simulink model "spacecraft_attitude_model"  (R2024b)
settings: Solver=ode4  StartTime=t0  StopTime=tf  FixedStep=0.1  RelTol=1e-3
values from neighbouring files (symbols this model uses):
  a = (((T/(2*pi))^2*mu_earth)^(1/3))    (= 7069867.85099)    [main_spacecraft_attitude_dynamics.m]
  A_body1 = surface(1)    [main_spacecraft_attitude_dynamics.m]
  A_body2 = surface(2)    [main_spacecraft_attitude_dynamics.m]
  A_body3 = surface(3)    [main_spacecraft_attitude_dynamics.m]
  A_body4 = surface(4)    [main_spacecraft_attitude_dynamics.m]
  A_body5 = surface(5)    [main_spacecraft_attitude_dynamics.m]
  A_body6 = surface(6)    [main_spacecraft_attitude_dynamics.m]
  A_panel1 = surface(7)    [main_spacecraft_attitude_dynamics.m]
  A_panel2 = surface(8)    [main_spacecraft_attitude_dynamics.m]
  A_panel3 = surface(9)    [main_spacecraft_attitude_dynamics.m]
  A_panel4 = surface(10)    [main_spacecraft_attitude_dynamics.m]
  alpha = [alpha1,alpha2,alpha3]    [main_spacecraft_attitude_dynamics.m]
  Ap = pinv(Ar)    [main_spacecraft_attitude_dynamics.m]
  Ar = Ar./norm(Ar)    [main_spacecraft_attitude_dynamics.m]
  AtmosphereModel = struct()    [AtmosphereData.m]    (also in main_spacecraft_attitude_dynamics.m)
  CD = 2.6    [main_spacecraft_attitude_dynamics.m]
  D_max = 50    [main_spacecraft_attitude_dynamics.m]
  Detumbling_time = 5000    [main_spacecraft_attitude_dynamics.m]
  e = 0.001    [main_spacecraft_attitude_dynamics.m]
  FOV = 128 * pi/180    (= 2.23402144255)    [main_spacecraft_attitude_dynamics.m]
  g1_0 = DGRF2020(1).g_nm    [main_spacecraft_attitude_dynamics.m]
  g1_1 = DGRF2020(2).g_nm    [main_spacecraft_attitude_dynamics.m]
  H = 700    [main_spacecraft_attitude_dynamics.m]
  h0 = 0    [main_spacecraft_attitude_dynamics.m]
  h1_1 = DGRF2020(2).h_nm    [main_spacecraft_attitude_dynamics.m]
  i = deg2rad(98.18)    [main_spacecraft_attitude_dynamics.m]
  Ir = 0.1    [main_spacecraft_attitude_dynamics.m]
  J = EXTRACTED_DATA.I_total    [main_spacecraft_attitude_dynamics.m]
  j_B = [0.01, 0.05, 0.01]'    [main_spacecraft_attitude_dynamics.m]
  k1 = max(max(kd_slew))    [main_spacecraft_attitude_dynamics.m]
  k2 = max(max(kp_slew))    [main_spacecraft_attitude_dynamics.m]
  Kw = max(max(kp_detumbling))    [main_spacecraft_attitude_dynamics.m]
  n = sqrt((G*M_E)/(r_earth^3))    [main_spacecraft_attitude_dynamics.m]
  N_B1 = N_B(1, :)'    [main_spacecraft_attitude_dynamics.m]
  N_B2 = N_B(2, :)'    [main_spacecraft_attitude_dynamics.m]
  N_B3 = N_B(3, :)'    [main_spacecraft_attitude_dynamics.m]
  N_B4 = N_B(4, :)'    [main_spacecraft_attitude_dynamics.m]
  N_B5 = N_B(5, :)'    [main_spacecraft_attitude_dynamics.m]
  N_B6 = N_B(6, :)'    [main_spacecraft_attitude_dynamics.m]
  N_P1 = N_B(7, :)'    [main_spacecraft_attitude_dynamics.m]
  N_P2 = N_B(8, :)'    [main_spacecraft_attitude_dynamics.m]
  N_P3 = N_B(9, :)'    [main_spacecraft_attitude_dynamics.m]
  N_P4 = N_B(10, :)'    [main_spacecraft_attitude_dynamics.m]
  n_S = (2*pi)/T_S    (= 1.99238499086e-07)    [main_spacecraft_attitude_dynamics.m]
  om = deg2rad(0)    [main_spacecraft_attitude_dynamics.m]
  P = Fe/c    (= 4.52980041279e-06)    [main_spacecraft_attitude_dynamics.m]
  pd_body1 = rho_D(1)    [main_spacecraft_attitude_dynamics.m]
  pd_body2 = rho_D(2)    [main_spacecraft_attitude_dynamics.m]
  pd_body3 = rho_D(3)    [main_spacecraft_attitude_dynamics.m]
  pd_body4 = rho_D(4)    [main_spacecraft_attitude_dynamics.m]
  pd_body5 = rho_D(5)    [main_spacecraft_attitude_dynamics.m]
  pd_body6 = rho_D(6)    [main_spacecraft_attitude_dynamics.m]
  pd_panel1 = rho_D(7)    [main_spacecraft_attitude_dynamics.m]
  pd_panel2 = rho_D(8)    [main_spacecraft_attitude_dynamics.m]
  pd_panel3 = rho_D(9)    [main_spacecraft_attitude_dynamics.m]
  pd_panel4 = rho_D(10)    [main_spacecraft_attitude_dynamics.m]
  ps_body1 = rho_S(1)    [main_spacecraft_attitude_dynamics.m]
  ps_body2 = rho_S(2)    [main_spacecraft_attitude_dynamics.m]
  ps_body3 = rho_S(3)    [main_spacecraft_attitude_dynamics.m]
  ps_body4 = rho_S(4)    [main_spacecraft_attitude_dynamics.m]
  ps_body5 = rho_S(5)    [main_spacecraft_attitude_dynamics.m]
  ps_body6 = rho_S(6)    [main_spacecraft_attitude_dynamics.m]
  ps_panel1 = rho_S(7)    [main_spacecraft_attitude_dynamics.m]
  ps_panel2 = rho_S(8)    [main_spacecraft_attitude_dynamics.m]
  ps_panel3 = rho_S(9)    [main_spacecraft_attitude_dynamics.m]
  ps_panel4 = rho_S(10)    [main_spacecraft_attitude_dynamics.m]
  q0 = [q1_0 q2_0 q3_0 q4_0]    [main_spacecraft_attitude_dynamics.m]
  r_earth = (R_earth + H)*10^3    (= 7078136.3)    [main_spacecraft_attitude_dynamics.m]
  R_earth = 6378.1363    [main_spacecraft_attitude_dynamics.m]
  r_f1 = r_F(1, :)'    [main_spacecraft_attitude_dynamics.m]
  r_f10 = r_F(10, :)'    [main_spacecraft_attitude_dynamics.m]
  r_f2 = r_F(2, :)'    [main_spacecraft_attitude_dynamics.m]
  r_f3 = r_F(3, :)'    [main_spacecraft_attitude_dynamics.m]
  r_f4 = r_F(4, :)'    [main_spacecraft_attitude_dynamics.m]
  r_f5 = r_F(5, :)'    [main_spacecraft_attitude_dynamics.m]
  r_f6 = r_F(6, :)'    [main_spacecraft_attitude_dynamics.m]
  r_f7 = r_F(7, :)'    [main_spacecraft_attitude_dynamics.m]
  r_f8 = r_F(8, :)'    [main_spacecraft_attitude_dynamics.m]
  r_f9 = r_F(9, :)'    [main_spacecraft_attitude_dynamics.m]
  r_Sun = 149597870    [main_spacecraft_attitude_dynamics.m]
  RAAN = deg2rad(RAAN)    [main_spacecraft_attitude_dynamics.m]
  sigma_b = RRW*(pi/180)*(1/3600)*(1/sqrt(Ts))    [main_spacecraft_attitude_dynamics.m]
  sigma_mag = 10^-6    (= 1e-06)    [main_spacecraft_attitude_dynamics.m]
  sigma_n = ARW*(pi/180)*(1/60)*(1/sqrt(Ts))    [main_spacecraft_attitude_dynamics.m]
  T_coil_max = 50 * 45*10^-6    (= 0.00225)    [main_spacecraft_attitude_dynamics.m]
  th0 = 0    [main_spacecraft_attitude_dynamics.m]
  v0 = [0 0 0]    [main_spacecraft_attitude_dynamics.m]
  variance_Ss = (a_sun)^2    (= 3.24)    [main_spacecraft_attitude_dynamics.m]
  w_0 = [-3, 3, 3]'    [main_spacecraft_attitude_dynamics.m]
  w_E = (2*pi)/(24*60*60)    (= 7.27220521664e-05)    [main_spacecraft_attitude_dynamics.m]
  w_LN = [0 0 0]'    [main_spacecraft_attitude_dynamics.m]
undefined symbols (not defined in the file or in its folder): A_Ss_orienation
libraries: matrix_library x38, slpidlib x2, aerolibutil x1, vrlib x1
(part 2 of 4)

== system spacecraft_attitude_model/Kinematics/quaternions to DCM ==
  note: Also here it should be A_NB 'cause we are going from
      | the inertial frame reference to the body one
  note: In reality it should be called A_BN but in the lab slides they call it in this way
  q : Inport
  To Workspace : ToWorkspace  VariableName=A_NB  SampleTime=-1
  q2A_DCM : Subsystem
  A_BN : Outport
  wires:
  q2A_DCM/1(A_NB) -> A_BN/1, To Workspace/1
  q/1 -> q2A_DCM/1(q)

== system spacecraft_attitude_model/Pointing error/DCM err (1) ==
  note: To wrap the acos
  A_ref : Inport
  Acos : Trigonometry  Operator=acos
  Constant : Constant
  Gain : Gain  Gain=180/pi
  Gain1 : Gain  Gain=0.5
  MATLAB Function : MATLAB Function  TreatAsAtomicUnit=on
  Saturation4 : Saturate  UpperLimit=1  LowerLimit=-1
  Sum : Sum  Inputs=-+|
  err : Outport
  wires:
  A_ref/1 -> MATLAB Function/1(A)
  Sum/1 -> Gain1/1
  Acos/1 -> Gain/1
  Constant/1 -> Sum/1
  Gain/1 -> err/1
  Gain1/1 -> Saturation4/1
  MATLAB Function/1(tr) -> Sum/2
  Saturation4/1 -> Acos/1

== system spacecraft_attitude_model/Pointing error/Subsystem1 ==
  note: q_BL = q_LN^-1 q_BN
  note: q_bn-1 q_LN v q_LN-1 q_BN
  q_BN_sensed : Inport
  q_LN : Inport  Port=2
  Gain1 : Gain  Gain=[-1; -1; -1; 1]
  Scope : Scope
  Scope1 : Scope
  Scope2 : Scope
  "q'' = q x q' " : Subsystem
  q_BL : Outport
  wires:
  "q'' = q x q' "/1(q'') -> q_BL/1  "q_BL"
  q_BN_sensed/1 -> Scope/1, "q'' = q x q' "/2(q')
  q_LN/1 -> Scope1/1, Gain1/1
  Gain1/1 -> Scope2/1, "q'' = q x q' "/1(q)  "q^-1"

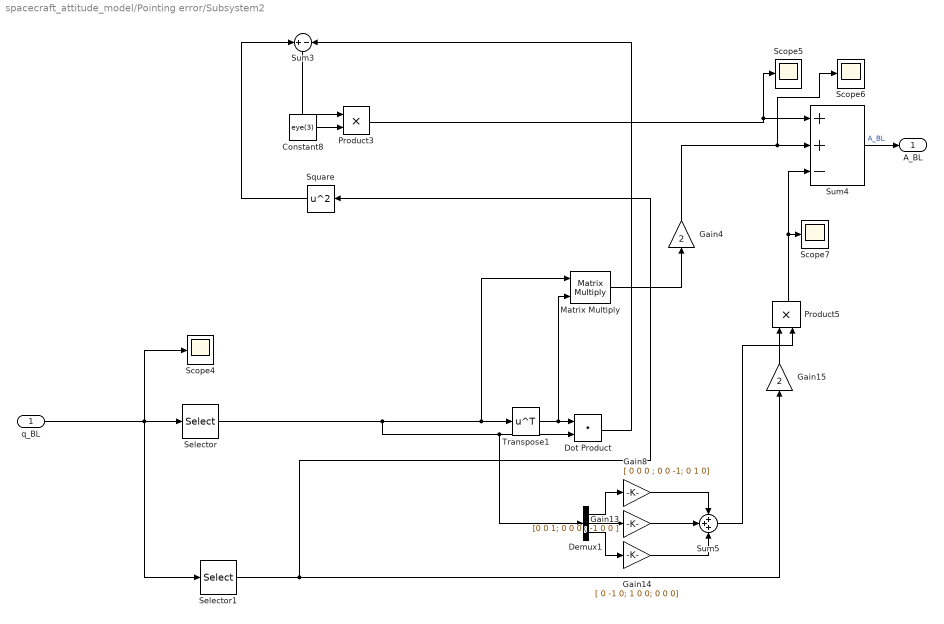
== system spacecraft_attitude_model/Pointing error/Subsystem2 ==
  q_BL : Inport
  Constant8 : Constant  Value=eye(3)
  Demux1 : Demux  Outputs=3
  Dot Product : DotProduct  OutDataTypeStr=Inherit: Inherit via internal rule
  Gain13 : Gain  Gain=[0 0 1; 0 0 0 ; -1 0 0 ]
  Gain14 : Gain  Gain=[ 0 -1 0; 1 0 0; 0 0 0]
  Gain15 : Gain  Gain=2
  Gain4 : Gain  Gain=2
  Gain8 : Gain  Gain=[ 0 0 0 ; 0 0 -1; 0 1 0]
  Matrix Multiply : Product  Multiplication=Matrix(*)
  Product3 : Product
  Product5 : Product
  Scope{4..7} (4 alike) : Scope
  Selector : Selector  NumberOfDimensions=2  InputPortWidth=3  IndexOptions=Index vector (dialog),Index vector (dialog)  Indices=[1 2 3],1  OutputSizes=1,1
  Selector1 : Selector  NumberOfDimensions=2  InputPortWidth=3  IndexOptions=Index vector (dialog),Index vector (dialog)  Indices=4,1  OutputSizes=1,1
  Square : Math  Operator=square
  Sum3 : Sum  Inputs=+-
  Sum4 : Sum  Inputs=++-
  Sum5 : Sum  Inputs=+++
  Transpose1 : Math  Operator=transpose
  A_BL : Outport
  wires:
  Constant8/1 -> Product3/2
  Matrix Multiply/1 -> Gain4/1
  Gain14/1 -> Sum5/3
  Product5/1 -> Scope7/1, Sum4/3
  Transpose1/1 -> Matrix Multiply/2, Dot Product/1
  Gain13/1 -> Sum5/2
  Sum5/1 -> Product5/2
  Gain8/1 -> Sum5/1
  Demux1/3 -> Gain14/1
  Sum4/1 -> A_BL/1  "A_BL"
  Product3/1 -> Scope5/1, Sum4/1
  Square/1 -> Sum3/1
  Selector/1 -> Matrix Multiply/1, Transpose1/1, Demux1/1, Dot Product/2
  Gain4/1 -> Scope6/1, Sum4/2
  Demux1/1 -> Gain8/1
  Gain15/1 -> Product5/1
  q_BL/1 -> Scope4/1, Selector/1, Selector1/1
  Sum3/1 -> Product3/1
  Dot Product/1 -> Sum3/2
  Selector1/1 -> Square/1, Gain15/1
  Demux1/2 -> Gain13/1

== system spacecraft_attitude_model/Pointing error/q_LN1 ==
  theta : Inport
  Constant : Constant  Value=[0; 0; 1]
  Constant1 : Constant  Value=[1; 0; 0]
  Constant2 : Constant  Value=i
  angle2quaternion : Subsystem
  angle2quaternion1 : Subsystem
  "q'' = q x q' " : Subsystem
  q_LN : Outport
  wires:
  theta/1 -> angle2quaternion/1(angle)
  Constant/1 -> angle2quaternion/2(e)
  Constant1/1 -> angle2quaternion1/2(e)
  Constant2/1 -> angle2quaternion1/1(angle)
  angle2quaternion1/1(q) -> "q'' = q x q' "/1(q)
  angle2quaternion/1(q) -> "q'' = q x q' "/2(q')
  "q'' = q x q' "/1(q'') -> q_LN/1

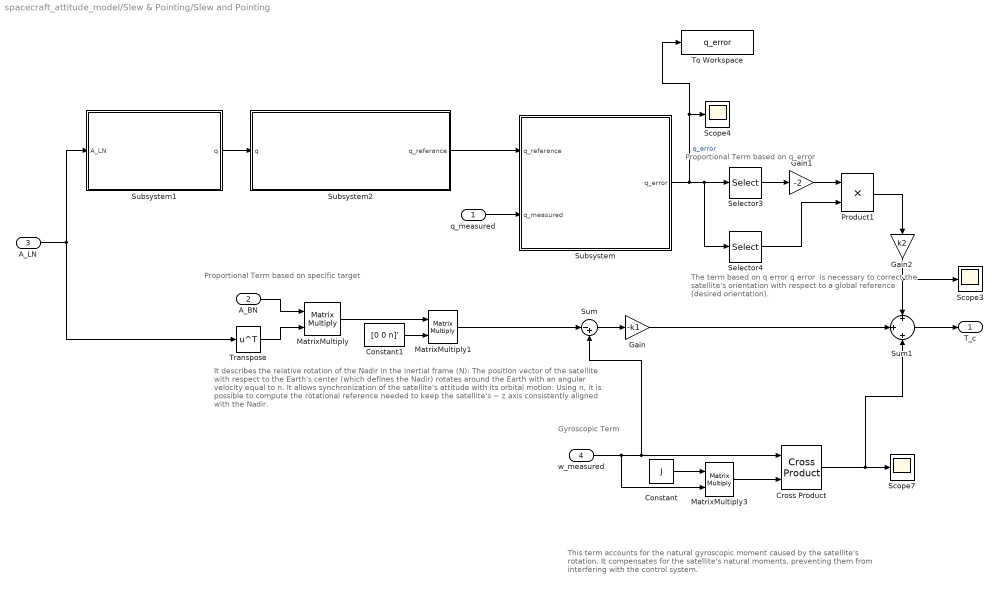
== system spacecraft_attitude_model/Slew & Pointing/Slew and Pointing ==
  note: The term based on q error q error ​ is necessary to correct the satellite's orientation with respect to a global reference (desired orientation).
  note: Proportional Term based on q_error
  note: This term accounts for the natural gyroscopic moment caused by the satellite's rotation. It compensates for the satellite's natural moments, preventing them from interfering with the control system.
  note: Proportional Term based on specific target
  note: It describes the relative rotation of the Nadir in the inertial frame (N): The position vector of the satellite with respect to the Earth's center (which defines the Nadir) rotates around the Earth with an angular velocity equal to n. It allows synchronization of the satellite's attitude with its orbital motion: Using n, it is possible to compute the rotational reference needed to keep the satellite's − z axis consistently aligned with the Nadir.
  note: Gyroscopic Term
  q_measured : Inport
  A_BN : Inport  Port=2
  A_LN : Inport  Port=3
  w_measured : Inport  Port=4
  Constant : Constant  Value=J
  Constant1 : Constant  Value=[0 0 n]'
  Cross Product : matrix_library/Cross Product
  Gain : Gain  Gain=-k1
  Gain1 : Gain  Gain=-2
  Gain2 : Gain  Gain=k2
  MatrixMultiply : Product  Multiplication=Matrix(*)
  MatrixMultiply1 : Product  Multiplication=Matrix(*)
  MatrixMultiply3 : Product  Multiplication=Matrix(*)
  Product1 : Product
  Scope3 : Scope
  Scope4 : Scope
  Scope7 : Scope
  Selector3 : Selector  InputPortWidth=4  IndexOptions=Index vector (dialog)  Indices=4  OutputSizes=1
  Selector4 : Selector  InputPortWidth=4  IndexOptions=Index vector (dialog)  Indices=[1:3]  OutputSizes=1
  Subsystem : Subsystem
  Subsystem1 : Subsystem
  Subsystem2 : Subsystem
  Sum : Sum  Inputs=|-+
  Sum1 : Sum  Inputs=+|+|+
  To Workspace : ToWorkspace  VariableName=q_error  SampleTime=-1
  Transpose : Math  Operator=transpose
  T_c : Outport
  wires:
  Transpose/1 -> MatrixMultiply/2
  MatrixMultiply/1 -> MatrixMultiply1/1
  w_measured/1 -> Sum/2, Cross Product/1, MatrixMultiply3/2
  Sum/1 -> Gain/1
  Gain/1 -> Sum1/2
  Constant/1 -> MatrixMultiply3/1
  MatrixMultiply3/1 -> Cross Product/2
  Cross Product/1 -> Scope7/1, Sum1/3
  Sum1/1 -> T_c/1
  q_measured/1 -> Subsystem/2(q_measured)
  Subsystem/1(q_error) -> Selector3/1, Selector4/1, To Workspace/1, Scope4/1  "q_error"
  Product1/1 -> Gain2/1
  Gain2/1 -> Sum1/1, Scope3/1
  Selector4/1 -> Product1/2
  Subsystem1/1(q) -> Subsystem2/1(q)
  A_BN/1 -> MatrixMultiply/1
  Subsystem2/1(q_referance) -> Subsystem/1(q_referance)
  Selector3/1 -> Gain1/1
  Gain1/1 -> Product1/1
  Constant1/1 -> MatrixMultiply1/2
  MatrixMultiply1/1 -> Sum/1
  A_LN/1 -> Subsystem1/1(A_LN), Transpose/1

== system spacecraft_attitude_model/Slew & Pointing/Subsystem ==
  b_measured : Inport
  T_control : Inport  Port=2
  w_measured : Inport  Port=3
  Constant : Constant  Value=Ar
  Inertia Wheel : Subsystem
  Magnetic coils : Subsystem
  Product : Product
  Scope : Scope  NumInputPorts=2
  Scope1 : Scope
  Subtract : Sum  Inputs=+-
  Sum : Sum  Inputs=|++
  To Workspace : ToWorkspace  VariableName=T_wheel_point1  SampleTime=-1
  T_act : Outport
  wires:
  Magnetic coils/1(T_coils) -> Sum/2
  Constant/1 -> Product/1
  Product/1 -> Subtract/2, Scope/1, Inertia Wheel/2(T_c_inertia)  "T_c_inertia"
  Inertia Wheel/1(T_wheel) -> To Workspace/1, Sum/1
  Sum/1 -> Scope1/1, T_act/1
  T_control/1 -> Product/2, Subtract/1
  Subtract/1 -> Magnetic coils/1(T_Control), Scope/2  "T_c_coils"
  b_measured/1 -> Magnetic coils/2(b_measured)
  w_measured/1 -> Inertia Wheel/1(w_measured)

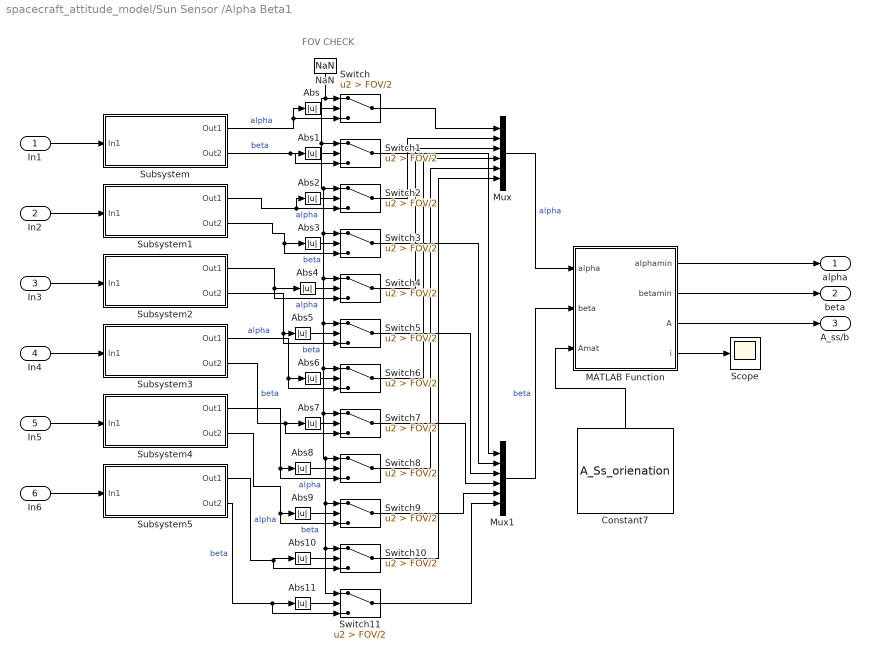
== system spacecraft_attitude_model/Sun Sensor /Alpha Beta1 ==
  note: FOV CHECK
  In1 : Inport
  In2 : Inport  Port=2
  In3 : Inport  Port=3
  In4 : Inport  Port=4
  In5 : Inport  Port=5
  In6 : Inport  Port=6
  Abs{,1..11} (12 alike) : Abs  SaturateOnIntegerOverflow=off
  Constant7 : Constant  Value=A_Ss_orienation
  MATLAB Function : MATLAB Function  TreatAsAtomicUnit=on
  Mux : Mux  Inputs=6
  Mux1 : Mux  Inputs=6
  NaN : Constant  Value=NaN  OutDataTypeStr=Inherit: Inherit via back propagation
  Scope : Scope
  Subsystem : Subsystem
  Subsystem1 : Subsystem
  Subsystem2 : Subsystem
  Subsystem3 : Subsystem
  Subsystem4 : Subsystem
  Subsystem5 : Subsystem
  Switch{,1..11} (12 alike) : Switch  Criteria=u2 > Threshold  Threshold=FOV/2  SaturateOnIntegerOverflow=off  InputSameDT=off
  alpha : Outport
  beta : Outport  Port=2
  A_ss/b : Outport  Port=3
  wires:
  Subsystem1/1(Out1) -> Abs2/1, Switch2/3  "alpha"
  Switch6/1 -> Mux/4
  Subsystem/2(Out2) -> Switch1/3, Abs1/1  "beta"
  In5/1 -> Subsystem4/1(In1)
  Abs10/1 -> Switch10/2
  Subsystem4/1(Out1) -> Switch8/3, Abs8/1  "alpha"
  Abs2/1 -> Switch2/2
  Subsystem2/1(Out1) -> Abs4/1, Switch4/3  "alpha"
  Subsystem3/1(Out1) -> Switch6/3, Abs6/1  "alpha"
  Switch1/1 -> Mux1/1
  Abs8/1 -> Switch8/2
  Switch5/1 -> Mux1/3
  Mux/1 -> MATLAB Function/1(alpha)  "alpha"
  Switch9/1 -> Mux1/5
  Subsystem2/2(Out2) -> Abs5/1, Switch5/3  "beta"
  Abs3/1 -> Switch3/2
  Subsystem1/2(Out2) -> Abs3/1, Switch3/3  "beta"
  Subsystem4/2(Out2) -> Switch9/3, Abs9/1  "beta"
  Switch11/1 -> Mux1/6
  Abs6/1 -> Switch6/2
  Switch3/1 -> Mux1/2
  Abs11/1 -> Switch11/2
  Abs1/1 -> Switch1/2
  In2/1 -> Subsystem1/1(In1)
  NaN/1 -> Switch11/1, Switch10/1, Switch9/1, Switch8/1, Switch7/1, Switch6/1, Switch5/1, Switch4/1, Switch3/1, Switch2/1, Switch1/1, Switch/1
  Subsystem/1(Out1) -> Abs/1, Switch/3  "alpha"
  Abs4/1 -> Switch4/2
  Subsystem3/2(Out2) -> Switch7/3, Abs7/1  "beta"
  Subsystem5/1(Out1) -> Switch10/3, Abs10/1  "alpha"
  Switch8/1 -> Mux/5
  Subsystem5/2(Out2) -> Abs11/1, Switch11/3  "beta"
  Switch7/1 -> Mux1/4
  In6/1 -> Subsystem5/1(In1)
  Abs9/1 -> Switch9/2
  Switch2/1 -> Mux/2
  Abs7/1 -> Switch7/2
  Abs5/1 -> Switch5/2
  Switch4/1 -> Mux/3
  Switch/1 -> Mux/1
  Abs/1 -> Switch/2
  Switch10/1 -> Mux/6
  In1/1 -> Subsystem/1(In1)
  Mux1/1 -> MATLAB Function/2(beta)  "beta"
  In4/1 -> Subsystem3/1(In1)
  In3/1 -> Subsystem2/1(In1)
  MATLAB Function/1(alphamin) -> alpha/1
  Constant7/1 -> MATLAB Function/3(Amat)
  MATLAB Function/4(i) -> Scope/1
  MATLAB Function/2(betamin) -> beta/1
  MATLAB Function/3(A) -> A_ss/b/1

== system spacecraft_attitude_model/Sun Sensor /Angle erros1 ==
  alpha_x : Inport
  alpha_y : Inport  Port=2
  alpha_z : Inport  Port=3
  Constant1 : Constant  Value=[1 0 0; 0 1 0; 0 0 1]
  Gain5 : Gain  Gain=[0 0 0; 0 0 1; 0 -1 0]
  Gain6 : Gain  Gain=[0 0 -1; 0 0 0; 1 0 0]
  Gain7 : Gain  Gain=[0 1 0; -1 0 0; 0 0 0]
  Sum : Sum  Inputs=|++++
  Out1 : Outport
  wires:
  Gain7/1 -> Sum/3
  alpha_y/1 -> Gain6/1
  Gain5/1 -> Sum/1
  alpha_x/1 -> Gain5/1
  Constant1/1 -> Sum/4
  Sum/1 -> Out1/1
  Gain6/1 -> Sum/2
  alpha_z/1 -> Gain7/1

== system spacecraft_attitude_model/Sun Sensor /Norm ==
  In1 : Inport
  Demux : Demux  Outputs=3
  Sqrt : Sqrt
  Square : Math  Operator=square
  Square1 : Math  Operator=square
  Square2 : Math  Operator=square
  Sum : Sum  Inputs=|+++
  Out1 : Outport
  wires:
  Demux/3 -> Square2/1
  In1/1 -> Demux/1
  Demux/1 -> Square/1
  Demux/2 -> Square1/1
  Square/1 -> Sum/1
  Square1/1 -> Sum/2
  Square2/1 -> Sum/3
  Sum/1 -> Sqrt/1
  Sqrt/1 -> Out1/1

== system spacecraft_attitude_model/Torque to w_dot_control/Torque to w_dot ==
  T_c : Inport
  Constant1 : Constant  Value=J
  Divide : Product  Inputs=*/  Multiplication=Matrix(*)
  "w_dot_control " : Outport
  wires:
  Divide/1 -> "w_dot_control "/1
  Constant1/1 -> Divide/2
  T_c/1 -> Divide/1

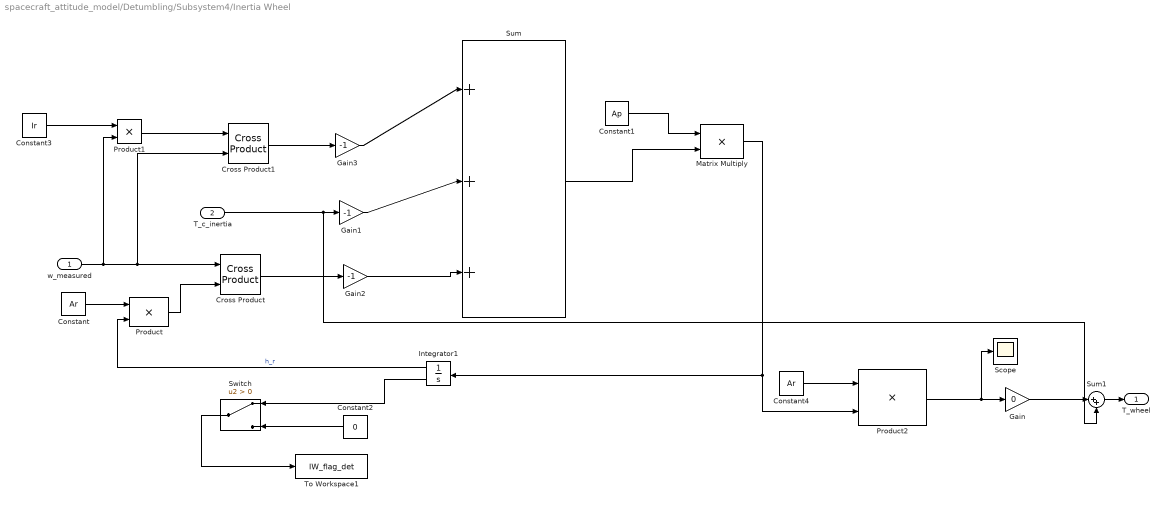
== system spacecraft_attitude_model/Detumbling/Subsystem4/Inertia Wheel ==
  w_measured : Inport
  T_c_inertia : Inport  Port=2
  Constant : Constant  Value=Ar
  Constant1 : Constant  Value=Ap
  Constant2 : Constant  Value=0
  Constant3 : Constant  Value=Ir
  Constant4 : Constant  Value=Ar
  Cross Product : matrix_library/Cross Product
  Cross Product1 : matrix_library/Cross Product
  Gain : Gain  Gain=0
  Gain1 : Gain  Gain=-1
  Gain2 : Gain  Gain=-1
  Gain3 : Gain  Gain=-1
  Integrator1 : Integrator  InitialCondition=h0  LimitOutput=on  UpperSaturationLimit=0.005  LowerSaturationLimit=-0.005  ShowSaturationPort=on
  Matrix Multiply : Product
  Product : Product
  Product1 : Product
  Product2 : Product
  Scope : Scope
  Sum : Sum  Inputs=|+++
  Sum1 : Sum  Inputs=|++
  Switch : Switch  Criteria=u2 > Threshold  SaturateOnIntegerOverflow=off  InputSameDT=off
  To Workspace1 : ToWorkspace  VariableName=IW_flag_det  SampleTime=-1
  T_wheel : Outport
  wires:
  Product/1 -> Cross Product/2
  Cross Product/1 -> Gain2/1
  w_measured/1 -> Product1/2, Cross Product1/2, Cross Product/1
  Gain2/1 -> Sum/3
  Constant1/1 -> Matrix Multiply/1
  Gain3/1 -> Sum/1
  Matrix Multiply/1 -> Product2/2, Integrator1/1
  Constant3/1 -> Product1/1
  Integrator1/1 -> Product/2  "h_r"
  Integrator1/2 -> Switch/1
  Constant2/1 -> Switch/3
  Constant/1 -> Product/1
  Product2/1 -> Scope/1, Gain/1
  Gain1/1 -> Sum/2
  Switch/1 -> To Workspace1/1
  Product1/1 -> Cross Product1/1
  Cross Product1/1 -> Gain3/1
  Constant4/1 -> Product2/1
  T_c_inertia/1 -> Sum1/2, Gain1/1
  Sum/1 -> Matrix Multiply/2
  Gain/1 -> Sum1/1
  Sum1/1 -> T_wheel/1

== system spacecraft_attitude_model/Detumbling/Subsystem4/Magnetic coils ==
  T_Control : Inport
  b_measured : Inport  Port=2
  Demux : Demux  Outputs=3
  Demux1 : Demux  Outputs=3
  Gain : Gain
  Gain1 : Gain
  Gain2 : Gain
  Norm1 : Subsystem
      settings: PortSchema="{\"entries\":[{\"content\":{\"sides\":[{\"content\":{},\"type\":\"ConnectorPlacement.EquallySpacedRectSide\",\"uuid\":\"c8e6b557-1f56-4290-9ece-bfc368650609\"},{\"content\":{\"connectorIds\":[\"Out1\"],\"side\":\"RIGHT\"},\"type\":\"ConnectorPlacement.EquallySpacedRectSide\",\"uuid\":\"77fa52b5-00ea-4466-8814-b89029d0f61f\"},{\"content\":{\"connectorIds\":[\"In1\"],\"side\":\"TOP\"},\"type\":\"ConnectorPlacement.EquallySpacedRectSide\",\"uuid\":\"5a1e965d-5eef-4834-963c-decfdd4da2be\"},{\"content\":{\"side\":\"BOTTOM\"},\"type\":\"ConnectorPlacement.EquallySpacedRectSide\",\"uuid\":\"d0b05173-3d81-4b7c-baba-8d47e4810e0f\"}]},\"type\":\"ConnectorPlacement.EquallySpacedConnector\",\"uuid\":\"bc13670f-664f-40fc-b4f3-9fab538d09d1\"}],\"packageUris\":[\"http://schema.mathworks.com/mf0/Connector/R2020b\"],\"version\":\"1.0\"}"
  Scope2 : Scope
  Square1 : Math  Operator=square
  Subsystem : Subsystem
  Subsystem1 : Subsystem
  Subsystem2 : Subsystem
  Vector Concatenate : Concatenate  NumInputs=3
  T_coils : Outport
  wires:
  Square1/1 -> Subsystem/3(b_norm^2), Subsystem1/3(b_norm^2), Subsystem2/3(b_norm^2)
  Demux1/2 -> Subsystem1/2(b_y)
  Demux/1 -> Gain/1
  Demux1/1 -> Subsystem/2(b_x)
  Gain1/1 -> Subsystem1/1(T_y)
  Gain/1 -> Subsystem/1(T_x)
  Gain2/1 -> Subsystem2/1(T_z)
  Demux1/3 -> Subsystem2/2(b_z)
  Demux/3 -> Gain2/1
  b_measured/1 -> Norm1/1(b), Demux1/1
  Norm1/1(b_norm) -> Square1/1  "b_norm"
  Demux/2 -> Gain1/1
  Vector Concatenate/1 -> T_coils/1, Scope2/1
  T_Control/1 -> Demux/1
  Subsystem2/1(T_coil_z) -> Vector Concatenate/3
  Subsystem1/1(T_coil_y) -> Vector Concatenate/2
  Subsystem/1(T_coil_x) -> Vector Concatenate/1

== system spacecraft_attitude_model/Disturbances Torque/Air Drag/A_Cross ==
  v_rB_versor : Inport
  A_CROSS1 : Subsystem
  A_CROSS10 : Subsystem
  A_CROSS2 : Subsystem
  A_CROSS3 : Subsystem
  A_CROSS4 : Subsystem
  A_CROSS5 : Subsystem
  A_CROSS6 : Subsystem
  A_CROSS7 : Subsystem
  A_CROSS8 : Subsystem
  A_CROSS9 : Subsystem
  A_cross1 : Outport
  A_cross2 : Outport  Port=2
  A_cross3 : Outport  Port=3
  A_cross4 : Outport  Port=4
  A_cross5 : Outport  Port=5
  A_cross6 : Outport  Port=6
  A_cross7 : Outport  Port=7
  A_cross8 : Outport  Port=8
  A_cross9 : Outport  Port=9
  A_cross10 : Outport  Port=10
  wires:
  A_CROSS5/1(A_cross2) -> A_cross5/1
  v_rB_versor/1 -> A_CROSS6/1(v_r_hat), A_CROSS7/1(v_r_hat), A_CROSS8/1(v_r_hat), A_CROSS9/1(v_r_hat), A_CROSS10/1(v_r_hat), A_CROSS5/1(v_r_hat), A_CROSS4/1(v_r_hat), A_CROSS3/1(v_r_hat), A_CROSS2/1(v_r_hat), A_CROSS1/1(v_r_hat)
  A_CROSS6/1(A_cross6) -> A_cross6/1
  A_CROSS4/1(A_cross4) -> A_cross4/1
  A_CROSS9/1(A_cross9) -> A_cross9/1
  A_CROSS2/1(A_cross2) -> A_cross2/1
  A_CROSS8/1(A_cross8) -> A_cross8/1
  A_CROSS3/1(A_cross3) -> A_cross3/1
  A_CROSS7/1(A_cross7) -> A_cross7/1
  A_CROSS10/1(A_cross10) -> A_cross10/1
  A_CROSS1/1(A_cross1) -> A_cross1/1

== system spacecraft_attitude_model/Disturbances Torque/Air Drag/Norm ==
  In1 : Inport
  Demux : Demux  Outputs=3
  Sqrt : Sqrt
  Square : Math  Operator=square
  Square1 : Math  Operator=square
  Square2 : Math  Operator=square
  Sum : Sum  Inputs=|+++
  v_rB_norm : Outport
  wires:
  Demux/3 -> Square2/1
  In1/1 -> Demux/1
  Demux/1 -> Square/1
  Demux/2 -> Square1/1
  Square/1 -> Sum/1
  Square1/1 -> Sum/2
  Square2/1 -> Sum/3
  Sum/1 -> Sqrt/1
  Sqrt/1 -> v_rB_norm/1

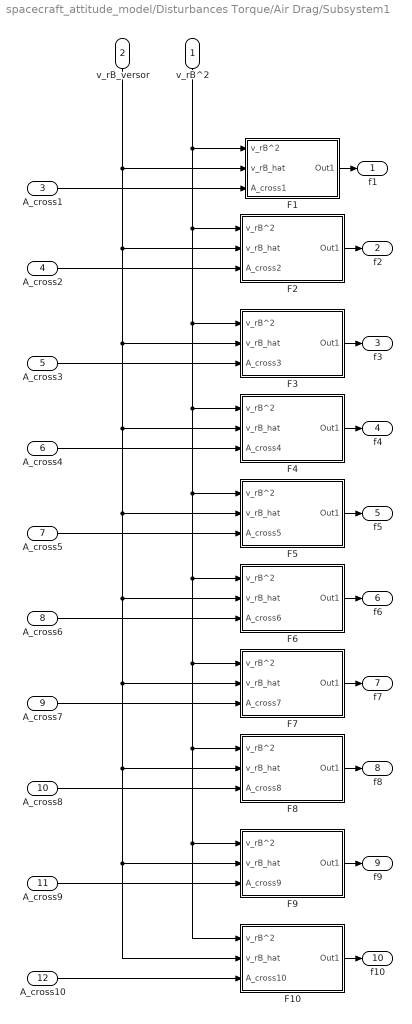
== system spacecraft_attitude_model/Disturbances Torque/Air Drag/Subsystem1 ==
  v_rB^2 : Inport
  v_rB_versor : Inport  Port=2
  A_cross1 : Inport  Port=3
  A_cross2 : Inport  Port=4
  A_cross3 : Inport  Port=5
  A_cross4 : Inport  Port=6
  A_cross5 : Inport  Port=7
  A_cross6 : Inport  Port=8
  A_cross7 : Inport  Port=9
  A_cross8 : Inport  Port=10
  A_cross9 : Inport  Port=11
  A_cross10 : Inport  Port=12
  F1 : Subsystem
  F10 : Subsystem
  F2 : Subsystem
  F3 : Subsystem
  F4 : Subsystem
  F5 : Subsystem
  F6 : Subsystem
  F7 : Subsystem
  F8 : Subsystem
  F9 : Subsystem
  f1 : Outport
  f2 : Outport  Port=2
  f3 : Outport  Port=3
  f4 : Outport  Port=4
  f5 : Outport  Port=5
  f6 : Outport  Port=6
  f7 : Outport  Port=7
  f8 : Outport  Port=8
  f9 : Outport  Port=9
  f10 : Outport  Port=10
  wires:
  v_rB^2/1 -> F1/1(v_rB^2), F2/1(v_rB^2), F3/1(v_rB^2), F4/1(v_rB^2), F5/1(v_rB^2), F6/1(v_rB^2), F7/1(v_rB^2), F8/1(v_rB^2), F9/1(v_rB^2), F10/1(v_rB^2)
  A_cross6/1 -> F6/3(A_cross6)
  v_rB_versor/1 -> F1/2(v_rB_hat), F2/2(v_rB_hat), F3/2(v_rB_hat), F4/2(v_rB_hat), F5/2(v_rB_hat), F6/2(v_rB_hat), F7/2(v_rB_hat), F8/2(v_rB_hat), F9/2(v_rB_hat), F10/2(v_rB_hat)
  A_cross5/1 -> F5/3(A_cross5)
  F5/1(Out1) -> f5/1
  A_cross4/1 -> F4/3(A_cross4)
  A_cross3/1 -> F3/3(A_cross3)
  A_cross9/1 -> F9/3(A_cross9)
  A_cross1/1 -> F1/3(A_cross1)
  F10/1(Out1) -> f10/1
  F7/1(Out1) -> f7/1
  A_cross8/1 -> F8/3(A_cross8)
  F6/1(Out1) -> f6/1
  F2/1(Out1) -> f2/1
  F3/1(Out1) -> f3/1
  F8/1(Out1) -> f8/1
  F1/1(Out1) -> f1/1
  A_cross10/1 -> F10/3(A_cross10)
  F4/1(Out1) -> f4/1
  F9/1(Out1) -> f9/1
  A_cross7/1 -> F7/3(A_cross7)
  A_cross2/1 -> F2/3(A_cross2)

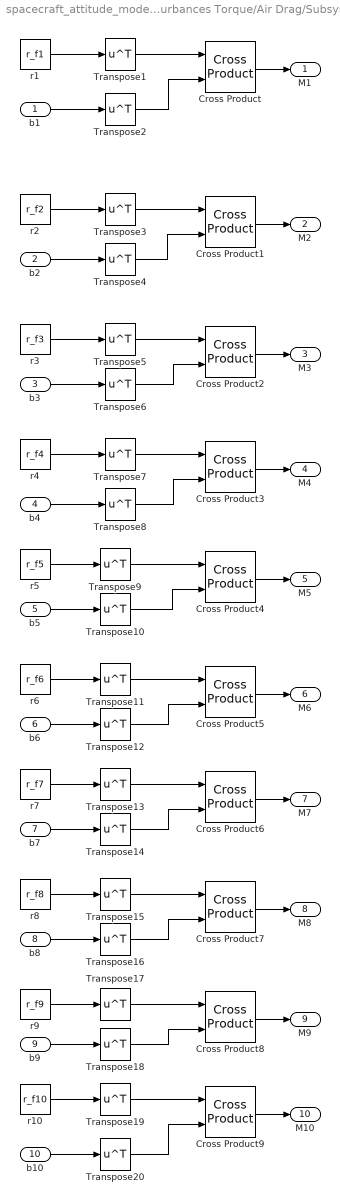
== system spacecraft_attitude_model/Disturbances Torque/Air Drag/Subsystem2 ==
  b1 : Inport
  b2 : Inport  Port=2
  b3 : Inport  Port=3
  b4 : Inport  Port=4
  b5 : Inport  Port=5
  b6 : Inport  Port=6
  b7 : Inport  Port=7
  b8 : Inport  Port=8
  b9 : Inport  Port=9
  b10 : Inport  Port=10
  Cross Product{,1..9} (10 alike) : matrix_library/Cross Product
  Transpose{1..20} (20 alike) : Math  Operator=transpose
  r1 : Constant  Value=r_f1
  r10 : Constant  Value=r_f10
  r2 : Constant  Value=r_f2
  r3 : Constant  Value=r_f3
  r4 : Constant  Value=r_f4
  r5 : Constant  Value=r_f5
  r6 : Constant  Value=r_f6
  r7 : Constant  Value=r_f7
  r8 : Constant  Value=r_f8
  r9 : Constant  Value=r_f9
  M1 : Outport
  M2 : Outport  Port=2
  M3 : Outport  Port=3
  M4 : Outport  Port=4
  M5 : Outport  Port=5
  M6 : Outport  Port=6
  M7 : Outport  Port=7
  M8 : Outport  Port=8
  M9 : Outport  Port=9
  M10 : Outport  Port=10
  wires:
  r1/1 -> Transpose1/1
  r10/1 -> Transpose19/1
  Cross Product8/1 -> M9/1
  r2/1 -> Transpose3/1
  Cross Product6/1 -> M7/1
  r6/1 -> Transpose11/1
  r5/1 -> Transpose9/1
  r9/1 -> Transpose17/1
  r7/1 -> Transpose13/1
  r4/1 -> Transpose7/1
  r8/1 -> Transpose15/1
  b6/1 -> Transpose12/1
  b2/1 -> Transpose4/1
  r3/1 -> Transpose5/1
  b1/1 -> Transpose2/1
  Cross Product3/1 -> M4/1
  b8/1 -> Transpose16/1
  Cross Product1/1 -> M2/1
  b5/1 -> Transpose10/1
  Cross Product7/1 -> M8/1
  b3/1 -> Transpose6/1
  Cross Product4/1 -> M5/1
  Cross Product2/1 -> M3/1
  Cross Product/1 -> M1/1
  Cross Product5/1 -> M6/1
  b10/1 -> Transpose20/1
  Cross Product9/1 -> M10/1
  b9/1 -> Transpose18/1
  b7/1 -> Transpose14/1
  b4/1 -> Transpose8/1
  Transpose1/1 -> Cross Product/1
  Transpose2/1 -> Cross Product/2
  Transpose3/1 -> Cross Product1/1
  Transpose4/1 -> Cross Product1/2
  Transpose5/1 -> Cross Product2/1
  Transpose6/1 -> Cross Product2/2
  Transpose7/1 -> Cross Product3/1
  Transpose8/1 -> Cross Product3/2
  Transpose9/1 -> Cross Product4/1
  Transpose10/1 -> Cross Product4/2
  Transpose11/1 -> Cross Product5/1
  Transpose12/1 -> Cross Product5/2
  Transpose13/1 -> Cross Product6/1
  Transpose14/1 -> Cross Product6/2
  Transpose15/1 -> Cross Product7/1
  Transpose16/1 -> Cross Product7/2
  Transpose17/1 -> Cross Product8/1
  Transpose18/1 -> Cross Product8/2
  Transpose19/1 -> Cross Product9/1
  Transpose20/1 -> Cross Product9/2

== system spacecraft_attitude_model/Disturbances Torque/Gravity Gradient/Gravity Gradient ==
  A_BL : Inport
  -3*n^2 : Gain  Gain=-3*(n^2)
  Constant4 : Constant  Value=J
  Constant5 : Constant  Value=inv(J)
  Cross Product2 : matrix_library/Cross Product
  Matrix Multiply : Product  Multiplication=Matrix(*)
  Matrix Multiply1 : Product  Multiplication=Matrix(*)
  c : Subsystem
  w_dot_GG : Outport
  wires:
  Constant5/1 -> Matrix Multiply1/1
  Cross Product2/1 -> Matrix Multiply1/2  "(Jc x c)"
  Matrix Multiply1/1 -> -3*n^2/1
  Matrix Multiply/1 -> Cross Product2/1
  Constant4/1 -> Matrix Multiply/1
  c/1(c) -> Cross Product2/2, Matrix Multiply/2
  A_BL/1 -> c/1(A_BL)
  -3*n^2/1 -> w_dot_GG/1

== system spacecraft_attitude_model/Disturbances Torque/Gravity Gradient/w_dot to torque ==
  w : Inport
  w_dot_GG : Inport  Port=2
  Constant : Constant  Value=J
  Cross Product : matrix_library/Cross Product
  Product : Product  Multiplication=Matrix(*)
  Transpose2 : Math  Operator=transpose
  Transpose3 : Math  Operator=transpose
  T_GG : Outport
  wires:
  Constant/1 -> Product/1
  w_dot_GG/1 -> Transpose2/1
  Product/1 -> Transpose3/1
  Cross Product/1 -> T_GG/1
  w/1 -> Product/2
  Transpose2/1 -> Cross Product/1
  Transpose3/1 -> Cross Product/2

== system spacecraft_attitude_model/Disturbances Torque/Solar_Radiation_Torque/Norm ==
  In1 : Inport
  Demux : Demux  Outputs=3
  Sqrt : Sqrt
  Square : Math  Operator=square
  Square1 : Math  Operator=square
  Square2 : Math  Operator=square
  Sum : Sum  Inputs=|+++
  Out1 : Outport
  wires:
  Demux/3 -> Square2/1
  In1/1 -> Demux/1
  Demux/1 -> Square/1
  Demux/2 -> Square1/1
  Square/1 -> Sum/1
  Square1/1 -> Sum/2
  Square2/1 -> Sum/3
  Sum/1 -> Sqrt/1
  Sqrt/1 -> Out1/1

== system spacecraft_attitude_model/Disturbances Torque/Solar_Radiation_Torque/SQR Force body 10 ==
  norm S_B : Inport
  -P*A : Gain  Gain=-P * A_panel4
  Constant : Constant  Value=N_P4
  Constant1 : Constant  Value=pd_panel4 * 2/3
  Constant2 : Constant  Value=0
  Constant3 : Constant  Value=r_f10
  Cross Product : matrix_library/Cross Product
  Dot Product : DotProduct  OutDataTypeStr=Inherit: Inherit via internal rule
  Gain1 : Gain  Gain=2*ps_panel4
  Gain2 : Gain  Gain=N_P4
  Gain3 : Gain  Gain=1-ps_panel4
  Product : Product
  Sum : Sum  Inputs=|++
  Sum1 : Sum  Inputs=|++
  Switch : Switch  Criteria=u2 > Threshold  SaturateOnIntegerOverflow=off  InputSameDT=off
  To Workspace : ToWorkspace  VariableName=T10  SampleTime=-1
  T10 : Outport
  wires:
  Gain2/1 -> Sum1/1
  Dot Product/1 -> Switch/2, Gain1/1, -P*A/1
  Switch/1 -> To Workspace/1, T10/1
  Product/1 -> Cross Product/2
  -P*A/1 -> Product/1
  Constant3/1 -> Cross Product/1
  Constant2/1 -> Switch/3
  Constant/1 -> Dot Product/2
  Sum/1 -> Gain2/1
  Gain3/1 -> Sum1/2
  Cross Product/1 -> Switch/1
  norm S_B/1 -> Gain3/1, Dot Product/1
  Sum1/1 -> Product/2
  Gain1/1 -> Sum/1
  Constant1/1 -> Sum/2

== system spacecraft_attitude_model/Disturbances Torque/Solar_Radiation_Torque/SQR Force body 6 ==
  norm S_B : Inport
  -P*A : Gain  Gain=-P * A_body6
  Constant : Constant  Value=N_B6
  Constant1 : Constant  Value=pd_body6 * 2/3
  Constant2 : Constant  Value=0
  Constant3 : Constant  Value=r_f6
  Cross Product : matrix_library/Cross Product
  Dot Product : DotProduct  OutDataTypeStr=Inherit: Inherit via internal rule
  Gain1 : Gain  Gain=2*ps_body6
  Gain2 : Gain  Gain=N_B6
  Gain3 : Gain  Gain=1-ps_body6
  Product : Product
  Sum : Sum  Inputs=|++
  Sum1 : Sum  Inputs=|++
  Switch : Switch  Criteria=u2 > Threshold  SaturateOnIntegerOverflow=off  InputSameDT=off
  To Workspace : ToWorkspace  VariableName=T6  SampleTime=-1
  T6 : Outport
  wires:
  Gain1/1 -> Sum/1
  Switch/1 -> To Workspace/1, T6/1
  -P*A/1 -> Product/1
  Constant1/1 -> Sum/2
  Constant/1 -> Dot Product/2
  Constant2/1 -> Switch/3
  norm S_B/1 -> Gain3/1, Dot Product/1
  Sum1/1 -> Product/2
  Cross Product/1 -> Switch/1
  Gain3/1 -> Sum1/2
  Sum/1 -> Gain2/1
  Dot Product/1 -> Switch/2, Gain1/1, -P*A/1
  Gain2/1 -> Sum1/1
  Product/1 -> Cross Product/2
  Constant3/1 -> Cross Product/1

== system spacecraft_attitude_model/Disturbances Torque/Solar_Radiation_Torque/SQR Force body 7 ==
  norm S_B : Inport
  -P*A : Gain  Gain=-P * A_panel1
  Constant : Constant  Value=N_P1
  Constant1 : Constant  Value=pd_panel1 * 2/3
  Constant2 : Constant  Value=0
  Constant3 : Constant  Value=r_f7
  Cross Product : matrix_library/Cross Product
  Dot Product : DotProduct  OutDataTypeStr=Inherit: Inherit via internal rule
  Gain1 : Gain  Gain=2*ps_panel1
  Gain2 : Gain  Gain=N_P1
  Gain3 : Gain  Gain=1-ps_panel1
  Product : Product
  Scope : Scope
  Sum : Sum  Inputs=|++
  Sum1 : Sum  Inputs=|++
  Switch : Switch  Criteria=u2 > Threshold  SaturateOnIntegerOverflow=off  InputSameDT=off
  To Workspace : ToWorkspace  VariableName=T7  SampleTime=-1
  T7 : Outport
  wires:
  Gain1/1 -> Sum/1
  Switch/1 -> To Workspace/1, Scope/1, T7/1
  -P*A/1 -> Product/1
  Constant1/1 -> Sum/2
  Constant/1 -> Dot Product/2
  Constant2/1 -> Switch/3
  norm S_B/1 -> Gain3/1, Dot Product/1
  Sum1/1 -> Product/2
  Cross Product/1 -> Switch/1
  Gain3/1 -> Sum1/2
  Sum/1 -> Gain2/1
  Dot Product/1 -> Switch/2, Gain1/1, -P*A/1
  Gain2/1 -> Sum1/1
  Product/1 -> Cross Product/2
  Constant3/1 -> Cross Product/1

== system spacecraft_attitude_model/Disturbances Torque/Solar_Radiation_Torque/SQR Force body 8 ==
  norm S_B : Inport
  -P*A : Gain  Gain=-P * A_panel2
  Constant : Constant  Value=N_P2
  Constant1 : Constant  Value=pd_panel2 * 2/3
  Constant2 : Constant  Value=0
  Constant3 : Constant  Value=r_f8
  Cross Product : matrix_library/Cross Product
  Dot Product : DotProduct  OutDataTypeStr=Inherit: Inherit via internal rule
  Gain1 : Gain  Gain=2*ps_panel2
  Gain2 : Gain  Gain=N_P2
  Gain3 : Gain  Gain=1-ps_panel2
  Product : Product
  Scope : Scope
  Sum : Sum  Inputs=|++
  Sum1 : Sum  Inputs=|++
  Switch : Switch  Criteria=u2 > Threshold  SaturateOnIntegerOverflow=off  InputSameDT=off
  To Workspace : ToWorkspace  VariableName=T8  SampleTime=-1
  T8 : Outport
  wires:
  Gain2/1 -> Sum1/1
  Dot Product/1 -> Switch/2, Gain1/1, -P*A/1
  Switch/1 -> To Workspace/1, Scope/1, T8/1
  Product/1 -> Cross Product/2
  -P*A/1 -> Product/1
  Constant3/1 -> Cross Product/1
  Constant2/1 -> Switch/3
  Constant/1 -> Dot Product/2
  Sum/1 -> Gain2/1
  Gain3/1 -> Sum1/2
  Cross Product/1 -> Switch/1
  norm S_B/1 -> Gain3/1, Dot Product/1
  Sum1/1 -> Product/2
  Gain1/1 -> Sum/1
  Constant1/1 -> Sum/2

== system spacecraft_attitude_model/Disturbances Torque/Solar_Radiation_Torque/SQR Force body 9 ==
  norm S_B : Inport
  -P*A : Gain  Gain=-P * A_panel3
  Constant : Constant  Value=N_P3
  Constant1 : Constant  Value=pd_panel3 * 2/3
  Constant2 : Constant  Value=0
  Constant3 : Constant  Value=r_f9
  Cross Product : matrix_library/Cross Product
  Dot Product : DotProduct  OutDataTypeStr=Inherit: Inherit via internal rule
  Gain1 : Gain  Gain=2*ps_panel3
  Gain2 : Gain  Gain=N_P3
  Gain3 : Gain  Gain=1-ps_panel3
  Product : Product
  Scope : Scope
  Sum : Sum  Inputs=|++
  Sum1 : Sum  Inputs=|++
  Switch : Switch  Criteria=u2 > Threshold  SaturateOnIntegerOverflow=off  InputSameDT=off
  To Workspace : ToWorkspace  VariableName=T9  SampleTime=-1
  T9 : Outport
  wires:
  Gain2/1 -> Sum1/1
  Dot Product/1 -> Switch/2, Gain1/1, -P*A/1
  Switch/1 -> To Workspace/1, Scope/1, T9/1
  Product/1 -> Cross Product/2
  -P*A/1 -> Product/1
  Constant3/1 -> Cross Product/1
  Constant2/1 -> Switch/3
  Constant/1 -> Dot Product/2
  Sum/1 -> Gain2/1
  Gain3/1 -> Sum1/2
  Cross Product/1 -> Switch/1
  norm S_B/1 -> Gain3/1, Dot Product/1
  Sum1/1 -> Product/2
  Gain1/1 -> Sum/1
  Constant1/1 -> Sum/2

== system spacecraft_attitude_model/Disturbances Torque/Solar_Radiation_Torque/SQR Torque body 4 ==
  norm S_B : Inport
  -P*A : Gain  Gain=-P*A_body4
  Constant : Constant  Value=N_B4
  Constant1 : Constant  Value=pd_body4 * 2/3
  Constant2 : Constant  Value=0
  Constant3 : Constant  Value=r_f4
  Cross Product : matrix_library/Cross Product
  Dot Product : DotProduct  OutDataTypeStr=Inherit: Inherit via internal rule
  Gain1 : Gain  Gain=2*ps_body4
  Gain2 : Gain  Gain=N_B4
  Gain3 : Gain  Gain=1-ps_body4
  Product : Product
  Sum : Sum  Inputs=|++
  Sum1 : Sum  Inputs=|++
  Switch : Switch  Criteria=u2 > Threshold  SaturateOnIntegerOverflow=off  InputSameDT=off
  To Workspace : ToWorkspace  VariableName=T4  SampleTime=-1
  T4 : Outport
  wires:
  Product/1 -> Cross Product/2
  Sum/1 -> Gain2/1
  norm S_B/1 -> Gain3/1, Dot Product/1
  Constant3/1 -> Cross Product/1
  Gain2/1 -> Sum1/1
  Gain1/1 -> Sum/1
  Constant1/1 -> Sum/2
  Sum1/1 -> Product/2
  Switch/1 -> To Workspace/1, T4/1
  Gain3/1 -> Sum1/2
  Constant2/1 -> Switch/3
  Cross Product/1 -> Switch/1
  -P*A/1 -> Product/1
  Dot Product/1 -> Switch/2, Gain1/1, -P*A/1
  Constant/1 -> Dot Product/2

== system spacecraft_attitude_model/Disturbances Torque/Solar_Radiation_Torque/SQR Torque body 5 ==
  norm S_B : Inport
  -P*A : Gain  Gain=-P * A_body5
  Constant : Constant  Value=N_B5
  Constant1 : Constant  Value=pd_body5 * 2/3
  Constant2 : Constant  Value=0
  Constant3 : Constant  Value=r_f5
  Cross Product : matrix_library/Cross Product
  Dot Product : DotProduct  OutDataTypeStr=Inherit: Inherit via internal rule
  Gain1 : Gain  Gain=2*ps_body5
  Gain2 : Gain  Gain=N_B5
  Gain3 : Gain  Gain=1-ps_body5
  Product : Product
  Sum : Sum  Inputs=|++
  Sum1 : Sum  Inputs=|++
  Switch : Switch  Criteria=u2 > Threshold  SaturateOnIntegerOverflow=off  InputSameDT=off
  To Workspace : ToWorkspace  VariableName=T5  SampleTime=-1
  T5 : Outport
  wires:
  Product/1 -> Cross Product/2
  Sum/1 -> Gain2/1
  norm S_B/1 -> Gain3/1, Dot Product/1
  Constant3/1 -> Cross Product/1
  Gain2/1 -> Sum1/1
  Gain1/1 -> Sum/1
  Constant1/1 -> Sum/2
  Sum1/1 -> Product/2
  Switch/1 -> To Workspace/1, T5/1
  Gain3/1 -> Sum1/2
  Constant2/1 -> Switch/3
  Cross Product/1 -> Switch/1
  -P*A/1 -> Product/1
  Dot Product/1 -> Switch/2, Gain1/1, -P*A/1
  Constant/1 -> Dot Product/2

== system spacecraft_attitude_model/Disturbances Torque/Solar_Radiation_Torque/SQR torque body 1 ==
  note: Switch: If the body is not illuminated
      | T = 0, in fact <0
  norm S_B : Inport
  -P*A : Gain  Gain=-P*A_body1
  Constant : Constant  Value=N_B1
  Constant1 : Constant  Value=pd_body1 * 2/3
  Constant2 : Constant  Value=0
  Constant3 : Constant  Value=r_f1
  Cross Product : matrix_library/Cross Product
  Dot Product : DotProduct  OutDataTypeStr=Inherit: Inherit via internal rule
  Gain1 : Gain  Gain=2*ps_body1
  Gain2 : Gain  Gain=N_B1
  Gain3 : Gain  Gain=1-ps_body1
  Product : Product
  Scope : Scope
  Sum : Sum  Inputs=|++
  Sum1 : Sum  Inputs=|++
  Switch : Switch  Criteria=u2 > Threshold  SaturateOnIntegerOverflow=off  InputSameDT=off
  To Workspace : ToWorkspace  VariableName=T1  SampleTime=-1
  T1 : Outport
  wires:
  norm S_B/1 -> Gain3/1, Dot Product/1
  Constant/1 -> Dot Product/2
  Dot Product/1 -> Switch/2, Gain1/1, -P*A/1
  Gain1/1 -> Sum/1
  Constant1/1 -> Sum/2
  Sum/1 -> Gain2/1
  Gain2/1 -> Sum1/1
  Gain3/1 -> Sum1/2
  -P*A/1 -> Product/1
  Sum1/1 -> Product/2
  Switch/1 -> To Workspace/1, Scope/1, T1/1
  Constant2/1 -> Switch/3
  Product/1 -> Cross Product/2
  Cross Product/1 -> Switch/1
  Constant3/1 -> Cross Product/1

== system spacecraft_attitude_model/Disturbances Torque/Solar_Radiation_Torque/SQR torque body 3 ==
  norm S_B : Inport
  -P*A : Gain  Gain=-P*A_body3
  Constant : Constant  Value=N_B3
  Constant1 : Constant  Value=pd_body3 * 2/3
  Constant2 : Constant  Value=0
  Constant3 : Constant  Value=r_f3
  Cross Product : matrix_library/Cross Product
  Dot Product : DotProduct  OutDataTypeStr=Inherit: Inherit via internal rule
  Gain1 : Gain  Gain=2*ps_body3
  Gain2 : Gain  Gain=N_B3
  Gain3 : Gain  Gain=1-ps_body3
  Product : Product
  Sum : Sum  Inputs=|++
  Sum1 : Sum  Inputs=|++
  Switch : Switch  Criteria=u2 > Threshold  SaturateOnIntegerOverflow=off  InputSameDT=off
  To Workspace : ToWorkspace  VariableName=T3  SampleTime=-1
  T3 : Outport
  wires:
  Product/1 -> Cross Product/2
  Sum/1 -> Gain2/1
  norm S_B/1 -> Gain3/1, Dot Product/1
  Constant3/1 -> Cross Product/1
  Gain2/1 -> Sum1/1
  Gain1/1 -> Sum/1
  Constant1/1 -> Sum/2
  Sum1/1 -> Product/2
  Switch/1 -> To Workspace/1, T3/1
  Gain3/1 -> Sum1/2
  Constant2/1 -> Switch/3
  Cross Product/1 -> Switch/1
  -P*A/1 -> Product/1
  Dot Product/1 -> Switch/2, Gain1/1, -P*A/1
  Constant/1 -> Dot Product/2

== system spacecraft_attitude_model/Disturbances Torque/Solar_Radiation_Torque/SQR torquw body 2 ==
  norm S_B : Inport
  -P*A : Gain  Gain=-P*A_body2
  Constant : Constant  Value=N_B2
  Constant1 : Constant  Value=pd_body2 * 2/3
  Constant2 : Constant  Value=0
  Constant3 : Constant  Value=r_f2
  Cross Product : matrix_library/Cross Product
  Dot Product : DotProduct  OutDataTypeStr=Inherit: Inherit via internal rule
  Gain1 : Gain  Gain=2*ps_body2
  Gain2 : Gain  Gain=N_B2
  Gain3 : Gain  Gain=1-ps_body2
  Product : Product
  Sum : Sum  Inputs=|++
  Sum1 : Sum  Inputs=|++
  Switch : Switch  Criteria=u2 > Threshold  SaturateOnIntegerOverflow=off  InputSameDT=off
  To Workspace : ToWorkspace  VariableName=T2  SampleTime=-1
  T2 : Outport
  wires:
  Switch/1 -> To Workspace/1, T2/1
  Sum/1 -> Gain2/1
  -P*A/1 -> Product/1
  Product/1 -> Cross Product/2
  Gain1/1 -> Sum/1
  Constant3/1 -> Cross Product/1
  Gain3/1 -> Sum1/2
  Cross Product/1 -> Switch/1
  Constant/1 -> Dot Product/2
  Dot Product/1 -> Switch/2, Gain1/1, -P*A/1
  Constant1/1 -> Sum/2
  Gain2/1 -> Sum1/1
  norm S_B/1 -> Gain3/1, Dot Product/1
  Sum1/1 -> Product/2
  Constant2/1 -> Switch/3

== system spacecraft_attitude_model/Envoirment/Model/Magnetic Field ==
  r_N : Inport
  H0 : Subsystem
  b_Ned : Subsystem
  m : Subsystem
  b_N : Outport
  wires:
  r_N/1 -> b_Ned/3(r_N)
  b_Ned/1(b_N) -> b_N/1
  m/1(m) -> b_Ned/1(m)
  H0/1(H_0) -> b_Ned/2(H_0)

== system spacecraft_attitude_model/Envoirment/Model/Sun_Direction ==
  Clock : Clock
  Constant : Constant  Value=n_S
  Constant1 : Constant  Value=eps
  Constant2 : Constant  Value=r_Sun
  Cos : Trigonometry  Operator=cos
  Cos1 : Trigonometry  Operator=cos
  Mux : Mux  Inputs=3
  Product{,1..5} (6 alike) : Product
  Scope : Scope
  Sin : Trigonometry
  Sin1 : Trigonometry
  To Workspace1 : ToWorkspace  VariableName=time  SampleTime=-1
  To Workspace2 : ToWorkspace  VariableName=S_N  SampleTime=-1
  S_N : Outport
  wires:
  Product2/1 -> Mux/2  "r*sin(n_S*t)*cos(eps)"
  Constant/1 -> Product/2
  Product4/1 -> Mux/3  "r*sin(n_S*t)*sin(eps)"
  Product/1 -> Sin/1, Cos/1  "n_S*t"
  Constant1/1 -> Cos1/1, Sin1/1
  Product5/1 -> Mux/1  "r*cos(n_S*t)"
  Cos/1 -> Product5/2
  Constant2/1 -> Product5/1, Product2/1, Product4/1
  Sin/1 -> Product1/1, Product3/1
  Cos1/1 -> Product1/2
  Clock/1 -> To Workspace1/1, Product/1
  Product1/1 -> Product2/2
  Sin1/1 -> Product3/2
  Product3/1 -> Product4/2
  Mux/1 -> To Workspace2/1, Scope/1, S_N/1

== system spacecraft_attitude_model/Envoirment/Two_Body_Keplerian_Dynamics/2BP ==
  (1-e^2)^(3/2) : Constant  Value=(1-e^2)^(3/2)
  Constant : Constant
  Constant1 : Constant  Value=e
  Constant2 : Constant  Value=n
  Cos : Trigonometry  Operator=cos
  Divide1 : Product  Inputs=*/
  Integrator : Integrator  InitialCondition=th0
  Product : Product
  Product5 : Product
  Scope : Scope
  Square : Math  Operator=square
  Sum : Sum  Inputs=|++
  Theta : Outport
  wires:
  Integrator/1 -> Theta/1, Cos/1, Scope/1  "Theta"
  (1-e^2)^(3/2)/1 -> Divide1/2
  Product5/1 -> Divide1/1
  Constant2/1 -> Product5/2
  Square/1 -> Product5/1
  Divide1/1 -> Integrator/1
  Constant1/1 -> Product/1
  Cos/1 -> Product/2
  Sum/1 -> Square/1  "1+ecos(th)"
  Product/1 -> Sum/2
  Constant/1 -> Sum/1

== system spacecraft_attitude_model/Envoirment/Two_Body_Keplerian_Dynamics/Subsystem ==
  Theta : Inport
  Constant1 : Constant
  Constant3 : Constant  Value=e
  Cos : Trigonometry  Operator=cos
  Divide : Product  Inputs=*/
  Product6 : Product
  Sum : Sum  Inputs=|++
  To Workspace : ToWorkspace  VariableName=r_N  SampleTime=-1
  a*(1-e^2) : Constant  Value=a*(1-(e^2))  VectorParams1D=off
  rN : Subsystem
  r_N : Outport
  wires:
  Cos/1 -> Product6/2
  a*(1-e^2)/1 -> Divide/1
  Sum/1 -> Divide/2  "(1+ecos(th))"
  Product6/1 -> Sum/2
  Constant3/1 -> Product6/1
  Constant1/1 -> Sum/1
  Theta/1 -> rN/2(Theta), Cos/1  "Theta"
  Divide/1 -> rN/1(r)  "r"
  rN/1(r_N) -> To Workspace/1, r_N/1

== system spacecraft_attitude_model/Kinematics/quaternions/Norm ==
  In1 : Inport
  Demux : Demux
  Sqrt : Sqrt
  Square{,1..3} (4 alike) : Math  Operator=square
  Sum : Sum  Inputs=|++++
  Out1 : Outport
  wires:
  Demux/3 -> Square2/1
  In1/1 -> Demux/1
  Demux/1 -> Square/1
  Demux/2 -> Square1/1
  Square/1 -> Sum/1
  Square1/1 -> Sum/2
  Square2/1 -> Sum/3
  Sum/1 -> Sqrt/1
  Sqrt/1 -> Out1/1
  Demux/4 -> Square3/1
  Square3/1 -> Sum/4

== system spacecraft_attitude_model/Kinematics/quaternions/Omega(t) ==
  In1 : Inport
  Constant{,1..2,4} (4 alike) : Constant  Value=0
  Demux : Demux  Outputs=3
  Gain{,1..5} (6 alike) : Gain  Gain=-1
  Matrix Concatenate : Concatenate  NumInputs=4  Mode=Multidimensional array  ConcatenateDimension=2
  Mux{,1..3} (4 alike) : Mux
  Transpose : matrix_library/Transpose
  Out1 : Outport
  wires:
  Mux1/1 -> Matrix Concatenate/2
  Constant/1 -> Mux/1
  Constant4/1 -> Mux1/2
  Mux/1 -> Matrix Concatenate/1
  In1/1 -> Demux/1
  Demux/3 -> Mux3/4, Gain1/1, Mux/2, Gain3/1
  Demux/2 -> Mux3/1, Mux1/4, Gain/1, Gain2/1
  Gain/1 -> Mux/3
  Demux/1 -> Gain5/1, Mux1/3, Mux/4, Gain4/1
  Gain1/1 -> Mux1/1
  Gain2/1 -> Mux2/2
  Constant1/1 -> Mux2/4
  Gain3/1 -> Mux2/3
  Gain4/1 -> Mux2/1
  Mux2/1 -> Matrix Concatenate/4
  Gain5/1 -> Mux3/2
  Constant2/1 -> Mux3/3
  Mux3/1 -> Matrix Concatenate/3
  Matrix Concatenate/1 -> Transpose/1
  Transpose/1 -> Out1/1

== system spacecraft_attitude_model/Kinematics/quaternions to DCM/q2A_DCM ==
  q : Inport
  Constant : Constant  Value=eye(3)
  Constant1 : Constant  Value=eye(3)
  Creation of q vector skew Matrix : Subsystem
  Demux : Demux
  Dot Product : DotProduct  OutDataTypeStr=Inherit: Inherit via internal rule
  Gain : Gain  Gain=2
  Gain1 : Gain  Gain=2
  Product : Product
  Product1 : Product  Inputs=3  Multiplication=Matrix(*)
  Product3 : Product
  Square : Math  Operator=square
  Sum : Sum  Inputs=|++-
  Sum1 : Sum  Inputs=|-+
  Transpose : Math  Operator=transpose
  Vector Concatenate : Concatenate  NumInputs=3
  A_NB : Outport
  wires:
  Square/1 -> Sum1/2
  Demux/3 -> Vector Concatenate/3
  Gain1/1 -> Product1/1
  Product3/1 -> Sum/2
  Constant1/1 -> Product1/3
  Product1/1 -> Sum/1
  Demux/1 -> Vector Concatenate/1
  Demux/4 -> Product/1, Square/1  "q4"
  q/1 -> Demux/1
  Vector Concatenate/1 -> Creation of q vector skew Matrix/1(q), Gain1/1, Transpose/1, Dot Product/2  "q vector"
  Sum/1 -> A_NB/1
  Product/1 -> Gain/1
  Demux/2 -> Vector Concatenate/2
  Constant/1 -> Product3/2
  Dot Product/1 -> Sum1/1
  Sum1/1 -> Product3/1
  Gain/1 -> Sum/3
  Creation of q vector skew Matrix/1("[q]^") -> Product/2  "[q]^"
  Transpose/1 -> Dot Product/1, Product1/2

== system spacecraft_attitude_model/Pointing error/Subsystem1/q'' = q x q'  ==
  q : Inport
  q' : Inport  Port=2
  Demux : Demux
  Gain : Gain  Gain=[1 0 0 0; 0 1 0 0; 0 0 1 0; 0 0 0 1]
  Gain1 : Gain  Gain=[0 1 0 0; -1 0 0 0; 0 0 0 1; 0 0 -1 0]
  Gain2 : Gain  Gain=[0 0 -1 0; 0 0 0 1; 1 0 0 0; 0 -1 0 0]
  Gain3 : Gain  Gain=[0 0 0 1; 0 0 1 0; 0 -1 0 0; -1 0 0 0]
  MatrixMultiply : Product  Multiplication=Matrix(*)
  Sum : Sum  Inputs=++++
  q'' : Outport
  wires:
  q'/1 -> Demux/1
  Demux/4 -> Gain/1
  Demux/3 -> Gain1/1
  Demux/2 -> Gain2/1
  Demux/1 -> Gain3/1
  Gain3/1 -> Sum/1
  Gain2/1 -> Sum/2
  Gain1/1 -> Sum/3
  Gain/1 -> Sum/4
  Sum/1 -> MatrixMultiply/1
  q/1 -> MatrixMultiply/2
  MatrixMultiply/1 -> q''/1  "4x1"

== system spacecraft_attitude_model/Pointing error/q_LN1/angle2quaternion ==
  angle : Inport
  e : Inport  Port=2
  Cos : Trigonometry  Operator=cos
  Demux : Demux  Outputs=3
  Display : Display
  Gain : Gain  Gain=0.5
  Mux : Mux
  Product : Product
  Product1 : Product
  Product2 : Product
  Sin : Trigonometry
  Square{,1..3} (4 alike) : Math  Operator=square
  Sum : Sum  Inputs=++++
  q : Outport
  wires:
  angle/1 -> Gain/1
  e/1 -> Demux/1
  Mux/1 -> q/1
  Product/1 -> Square/1, Mux/1
  Product1/1 -> Square1/1, Mux/2
  Product2/1 -> Square2/1, Mux/3
  Cos/1 -> Square3/1, Mux/4
  Demux/1 -> Product/1
  Gain/1 -> Cos/1, Sin/1
  Sin/1 -> Product2/2, Product1/2, Product/2
  Demux/2 -> Product1/1
  Demux/3 -> Product2/1
  Square/1 -> Sum/1
  Square1/1 -> Sum/2
  Square2/1 -> Sum/3
  Square3/1 -> Sum/4
  Sum/1 -> Display/1

== system spacecraft_attitude_model/Pointing error/q_LN1/angle2quaternion1 ==
  note: 1
  angle : Inport
  e : Inport  Port=2
  Cos : Trigonometry  Operator=cos
  Demux : Demux  Outputs=3
  Display : Display
  Gain : Gain  Gain=0.5
  Mux : Mux
  Product : Product
  Product1 : Product
  Product2 : Product
  Sin : Trigonometry
  Square{,1..3} (4 alike) : Math  Operator=square
  Sum : Sum  Inputs=++++
  q : Outport
  wires:
  Sum/1 -> Display/1
  Square3/1 -> Sum/4
  Square2/1 -> Sum/3
  Square1/1 -> Sum/2
  Square/1 -> Sum/1
  Demux/3 -> Product2/1
  Demux/2 -> Product1/1
  Sin/1 -> Product/2, Product1/2, Product2/2
  Gain/1 -> Sin/1, Cos/1
  Demux/1 -> Product/1
  Cos/1 -> Mux/4, Square3/1
  Product2/1 -> Mux/3, Square2/1
  Product1/1 -> Mux/2, Square1/1
  Product/1 -> Mux/1, Square/1
  Mux/1 -> q/1
  e/1 -> Demux/1
  angle/1 -> Gain/1

== system spacecraft_attitude_model/Pointing error/q_LN1/q'' = q x q'  ==
  q : Inport
  q' : Inport  Port=2
  Demux : Demux
  Gain : Gain  Gain=[1 0 0 0; 0 1 0 0; 0 0 1 0; 0 0 0 1]
  Gain1 : Gain  Gain=[0 1 0 0; -1 0 0 0; 0 0 0 1; 0 0 -1 0]
  Gain2 : Gain  Gain=[0 0 -1 0; 0 0 0 1; 1 0 0 0; 0 -1 0 0]
  Gain3 : Gain  Gain=[0 0 0 1; 0 0 1 0; 0 -1 0 0; -1 0 0 0]
  MatrixMultiply : Product  Multiplication=Matrix(*)
  Sum : Sum  Inputs=++++
  q'' : Outport
  wires:
  q'/1 -> Demux/1
  Demux/4 -> Gain/1
  Demux/3 -> Gain1/1
  Demux/2 -> Gain2/1
  Demux/1 -> Gain3/1
  Gain3/1 -> Sum/1
  Gain2/1 -> Sum/2
  Gain1/1 -> Sum/3
  Gain/1 -> Sum/4
  Sum/1 -> MatrixMultiply/1
  q/1 -> MatrixMultiply/2
  MatrixMultiply/1 -> q''/1  "4x1"
